simulink model "AccTarSel"  (R2018b)
settings: Solver=FixedStepDiscrete  StartTime=0.0  StopTime=inf  FixedStep=0.01  RelTol=1e-3
PostLoadFcn:
  | if any(exist('dsrtsu_mdlpostloadfcn', 'file') ~= 0), dsrtsu_mdlpostloadfcn('Execute', bdroot); end
values from neighbouring files (symbols this model uses):
  P_adtMaxBDC = 1.0    [AccTarSel.sldd]
  P_aFOCApproachIntpAcitve = -0.6    [AccTarSel.sldd]
  P_aFOCApproachIntpEnsure = -1.8    [AccTarSel.sldd]
  P_CutInEnable = 1.0    [AccTarSel.sldd]
  P_dAimMin = 4.5    [AccTarSel.sldd]
  P_dAimMinAVP = 1.5    [AccTarSel.sldd]
  P_dObjDrvOffMax = 5.0    [AccTarSel.sldd]
  P_dObjDrvOffMin = 3.0    [AccTarSel.sldd]
  P_dObjLowHystDecToStop = 4.5    [AccTarSel.sldd]
  P_dObjLowHystDecToStopAVP = 1.5    [AccTarSel.sldd]
  P_dObjUpperHystDecToStop = 5.0    [AccTarSel.sldd]
  P_dResMax = 5.0    [AccTarSel.sldd]
  P_dStandStill = 3.0    [AccTarSel.sldd]
  P_dStandStillMin = 2.0    [AccTarSel.sldd]
  P_dvarYMax4PO = 1.0    [AccTarSel.sldd]
  P_dyCutInThres = 3.6    [AccTarSel.sldd]
  P_facBDCInit = 0.7    [AccTarSel.sldd]
  P_facBDCIterCalc = 0.8    [AccTarSel.sldd]
  P_facFOCNegDiff = 0.3    [AccTarSel.sldd]
  P_facFOCPosDiff = 0.2    [AccTarSel.sldd]
  P_kapHystThres = 0.0005    [AccTarSel.sldd]
  P_PlausIntegDisable = 0.0    [AccTarSel.sldd]
  P_plausMin4PO = 0.5    [AccTarSel.sldd]
  P_probExistMin4PO = 0.8    [AccTarSel.sldd]
  P_StandObjEnable = 0.0    [AccTarSel.sldd]
  P_tAxTrackNegLower = 0.3    [AccTarSel.sldd]
  P_tAxTrackNegUpper = 0.6    [AccTarSel.sldd]
  P_tAxTrackPosLower = 1.0    [AccTarSel.sldd]
  P_tAxTrackPosUpper = 2.0    [AccTarSel.sldd]
  P_tBDCStartFilt = 0.2    [AccTarSel.sldd]
  P_tCSC = 3.5    [AccTarSel.sldd]
  P_tCurvFilt = 0.2    [AccTarSel.sldd]
  P_tCutInFilt = 0.5    [AccTarSel.sldd]
  P_tFiltAxAbsPONegFast = 0.1    [AccTarSel.sldd]
  P_tFiltAxAbsPONegSlow = 0.4    [AccTarSel.sldd]
  P_tFiltAxAbsPOPosFast = 1.2    [AccTarSel.sldd]
  P_tFiltAxAbsPOPosSlow = 2.0    [AccTarSel.sldd]
  P_tFiltAxAbsPOStand = 2.0    [AccTarSel.sldd]
  P_tFiltDAim = 0.1    [AccTarSel.sldd]
  P_tFiltDsd = 0.1    [AccTarSel.sldd]
  P_tFiltSpdLim = 3.0    [AccTarSel.sldd]
  P_tFiltVxAxPOFast = 0.15    [AccTarSel.sldd]
  P_tFiltVxAxPOSlow = 0.25    [AccTarSel.sldd]
  P_tFOCStatAccelFast = 4.0    [AccTarSel.sldd]
  P_tFOCStatAccelSlow = 3.5    [AccTarSel.sldd]
  P_tFOCStatDecelFast = 4.0    [AccTarSel.sldd]
  P_tFOCStatDecelSlow = 3.2    [AccTarSel.sldd]
  P_tMinDrvPhase = 2.0    [AccTarSel.sldd]
  P_tPredObjLeav = 1.2    [AccTarSel.sldd]
  P_tRollingFilt = 0.5    [AccTarSel.sldd]
  P_tRollingFinFilt = 1.0    [AccTarSel.sldd]
  P_tSSCNeg = 4.5    [AccTarSel.sldd]
  P_tSSCPos = 5.5    [AccTarSel.sldd]
  P_tToStop = 5.0    [AccTarSel.sldd]
  P_tToStopInBDC = 6.0    [AccTarSel.sldd]
  P_tToStopTrig = 4.0    [AccTarSel.sldd]
  P_vEgoDecToStop = 3.0    [AccTarSel.sldd]
  P_vEgoLowBDC = 4.0    [AccTarSel.sldd]
  P_vFOCNegDiff = 4.0    [AccTarSel.sldd]
  P_vFOCPosDiff = 5.0    [AccTarSel.sldd]
  P_vFOCStationaryFast = 15.0    [AccTarSel.sldd]
  P_vFOCStationarySlow = 5.0    [AccTarSel.sldd]
  P_vObjDrvOff = 0.5    [AccTarSel.sldd]
  P_vObjLowHystDecToStop = 0.5    [AccTarSel.sldd]
  P_vObjNoStop = 1.0    [AccTarSel.sldd]
  P_vObjReCalc = 1.0    [AccTarSel.sldd]
  P_vObjStop = 0.3    [AccTarSel.sldd]
  P_vObjUpperHystDecToStop = 0.8    [AccTarSel.sldd]
  P_vStandStill = 0.3    [AccTarSel.sldd]
  P_vStandStillHyst = 0.3    [AccTarSel.sldd]
  P_vyCutInThres = 0.5    [AccTarSel.sldd]
libraries: simulink x21, LPFilter x12
(part 5 of 11)

== system AccTarSel/calcCancelFlag/If Action Subsystem1 ==
  SYS_Info : Inport
  HoldTimeK1 : Inport  Port=2
  Action Port : ActionPort  ActionType=elseif
  Add : Sum  Inputs=+-
  Bus Selector : BusSelector  OutputSignals=dT
  Constant : Constant  OutDataTypeStr=boolean
  Constant1 : Constant  Value=0  OutDataTypeStr=single
  Max : MinMax  Function=max  Inputs=2
  CancelFlag : Outport
  HoldTime : Outport  Port=2
  wires:
  Max/1 -> HoldTime/1
  Constant/1 -> CancelFlag/1
  SYS_Info/1 -> Bus Selector/1
  HoldTimeK1/1 -> Add/1
  Bus Selector/1 -> Add/2  "<dT>"
  Add/1 -> Max/1
  Constant1/1 -> Max/2

== system AccTarSel/calcCancelFlag/If Action Subsystem2 ==
  Action Port : ActionPort  ActionType=else
  Constant : Constant  Value=0  OutDataTypeStr=boolean
  Constant1 : Constant  Value=0  OutDataTypeStr=single
  CancelFlag : Outport
  HoldTime : Outport  Port=2
  wires:
  Constant/1 -> CancelFlag/1
  Constant1/1 -> HoldTime/1

== system AccTarSel/ACC_Control/AccelBoundCtrl/LowerLimitation ==
  note: expand lower limitation according to:
      | vehicle speed
      | slope
  Constant : Constant  Value=-5  OutDataTypeStr=single
  Out1 : Outport
  wires:
  Constant/1 -> Out1/1

== system AccTarSel/ACC_Control/AccelBoundCtrl/UpperLimitation ==
  note: expand lower limitation according to:
      | vehicle speed
      | slope
      | engine capacity
  Constant : Constant  Value=2  OutDataTypeStr=single
  Out1 : Outport
  wires:
  Constant/1 -> Out1/1

== system AccTarSel/ACC_Control/ArbitraryMix/Subsystem ==
  aCvArray : Inport
  numASrc : Inport  Port=2
  Add : Sum
  Constant : Constant  Value=0  OutDataTypeStr=int32
  Constant1 : Constant  Value=16  OutDataTypeStr=single
  Constant2 : Constant  OutDataTypeStr=int32
  For Iterator : ForIterator  IterationSource=external  IndexMode=Zero-based
  Memory : Memory  InheritSampleTime=on
  Memory1 : Memory  InheritSampleTime=on
  Relational Operator : RelationalOperator  Operator===  OutDataTypeStr=boolean  RndMeth=Simplest
  Relational Operator1 : RelationalOperator  Operator=<  OutDataTypeStr=boolean  RndMeth=Simplest
  Selector : Selector  IndexMode=Zero-based  InputPortWidth=4  IndexOptions=Index vector (port)  Indices=[1 3]  OutputSizes=1
  Switch : Switch  Criteria=u2 > Threshold
  Switch1 : Switch  Criteria=u2 > Threshold
  Switch2 : Switch  Criteria=u2 > Threshold
  aMin : Outport
  CMDType : Outport  Port=2
  wires:
  numASrc/1 -> For Iterator/1
  For Iterator/1 -> Selector/2, Add/1, Relational Operator/1
  Constant/1 -> Relational Operator/2
  Relational Operator/1 -> Switch/2
  Constant1/1 -> Switch/1
  aCvArray/1 -> Selector/1
  Selector/1 -> Switch1/1, Relational Operator1/1
  Switch/1 -> Switch1/3, Relational Operator1/2
  Memory/1 -> Switch/3
  Relational Operator1/1 -> Switch1/2, Switch2/2
  Switch1/1 -> aMin/1, Memory/1
  Switch2/1 -> Memory1/1, CMDType/1
  Memory1/1 -> Switch2/3
  Constant2/1 -> Add/2
  Add/1 -> Switch2/1

== system AccTarSel/ACC_Control/ArbitraryMix/calcAFOC ==
  FOCInfo : Inport
  Constant2 : Constant  Value=6  OutDataTypeStr=int32
  For Iterator Subsystem : Subsystem  TreatAsAtomicUnit=on
  Min : MinMax
  OR : Logic  Operator=OR  Inputs=1  AllPortsSameDT=off  OutDataTypeStr=boolean
  aFOC : Outport
  DecToStop : Outport  Port=2
  wires:
  Min/1 -> aFOC/1
  FOCInfo/1 -> For Iterator Subsystem/2(FOCInfo)
  For Iterator Subsystem/1(aFOCArray) -> Min/1
  For Iterator Subsystem/2(DecToStopArray) -> OR/1
  OR/1 -> DecToStop/1
  Constant2/1 -> For Iterator Subsystem/1(numFOC)

== system AccTarSel/ACC_Control/FollowObjCtrl/FollowObjInvalid ==
  Action Port : ActionPort  ActionType=else
  Constant : Constant  Value=16  OutDataTypeStr=single
  Constant1 : Constant  Value=0  OutDataTypeStr=boolean
  Constant{3..8,10} (7 alike) : Constant  Value=0  OutDataTypeStr=single
  Constant2 : Constant  OutDataTypeStr=boolean
  Constant9 : Constant  Value=0  OutDataTypeStr=boolean
  a : Outport
  DecToStop : Outport  Port=2
  FirstCyc : Outport  Port=3  InitialOutput=0
  dAim : Outport  Port=4  InitialOutput=0
  aStat : Outport  Port=5  InitialOutput=0
  aApproach : Outport  Port=6  InitialOutput=0
  ApproachCase : Outport  Port=7  InitialOutput=0
  tObjStop : Outport  Port=8  InitialOutput=0
  dSlowDown : Outport  Port=9  InitialOutput=0
  ObjLeaving : Outport  Port=10  InitialOutput=0
  dImmerseAdj : Outport  Port=11  InitialOutput=0
  wires:
  Constant/1 -> a/1
  Constant1/1 -> DecToStop/1
  Constant2/1 -> FirstCyc/1
  Constant3/1 -> dAim/1
  Constant4/1 -> aStat/1
  Constant5/1 -> aApproach/1
  Constant6/1 -> ApproachCase/1
  Constant7/1 -> tObjStop/1
  Constant8/1 -> dSlowDown/1
  Constant9/1 -> ObjLeaving/1
  Constant10/1 -> dImmerseAdj/1

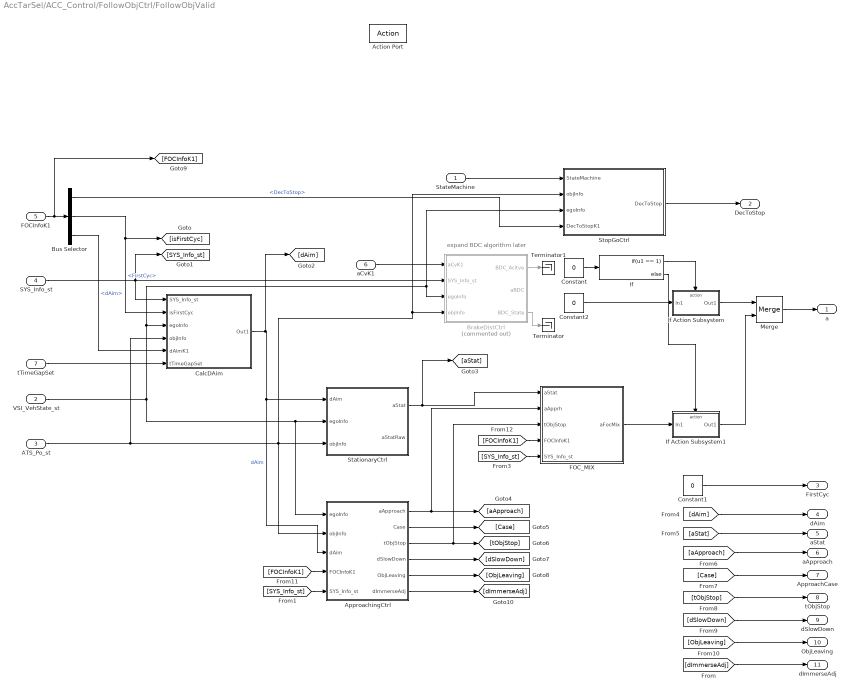
== system AccTarSel/ACC_Control/FollowObjCtrl/FollowObjValid ==
  note: expand BDC algorithm later
  StateMachine : Inport
  VSI_VehState_st : Inport  Port=2
  ATS_Po_st : Inport  Port=3
  SYS_Info_st : Inport  Port=4
  FOCInfoK1 : Inport  Port=5
  aCvK1 : Inport  Port=6
  tTimeGapSet : Inport  Port=7
  Action Port : ActionPort  ActionType=then
  ApproachingCtrl : Subsystem
  BrakeDistCtrl : Subsystem  Commented=on
  Bus Selector : BusSelector  OutputSignals=DecToStop,FirstCyc,dAim
  CalcDAim : Subsystem
  Constant : Constant  Value=0  OutDataTypeStr=boolean
  Constant1 : Constant  Value=0  OutDataTypeStr=boolean
  Constant2 : Constant  Value=0  OutDataTypeStr=single
  FOC_MIX : Subsystem
  If : If  IfExpression=u1 == 1
  If Action Subsystem : Subsystem  TreatAsAtomicUnit=on
  If Action Subsystem1 : Subsystem  TreatAsAtomicUnit=on
  Merge : Merge  InitialOutput=0
  StationaryCtrl : Subsystem
  StopGoCtrl : Subsystem
  Terminator : Terminator
  Terminator1 : Terminator
  a : Outport  InitialOutput=0
  DecToStop : Outport  Port=2  InitialOutput=0
  FirstCyc : Outport  Port=3  InitialOutput=0
  dAim : Outport  Port=4  InitialOutput=0
  aStat : Outport  Port=5  InitialOutput=0
  aApproach : Outport  Port=6  InitialOutput=0
  ApproachCase : Outport  Port=7  InitialOutput=0
  tObjStop : Outport  Port=8  InitialOutput=0
  dSlowDown : Outport  Port=9  InitialOutput=0
  ObjLeaving : Outport  Port=10  InitialOutput=0
  dImmerseAdj : Outport  Port=11  InitialOutput=0
  wires:
  ATS_Po_st/1 -> CalcDAim/4(objInfo), StopGoCtrl/2(objInfo), BrakeDistCtrl/4(objInfo), ApproachingCtrl/2(objInfo), StationaryCtrl/3(objInfo)
  CalcDAim/1(Out1) -> [dAim], ApproachingCtrl/3(dAim), StationaryCtrl/1(dAim)  "dAim"
  VSI_VehState_st/1 -> StopGoCtrl/3(egoInfo), BrakeDistCtrl/3(egoInfo), CalcDAim/3(egoInfo), ApproachingCtrl/1(egoInfo), StationaryCtrl/2(egoInfo)
  StationaryCtrl/1(aStat) -> [aStat], FOC_MIX/1(aStat)
  ApproachingCtrl/1(aApproach) -> [aApproach], FOC_MIX/2(aApprh)
  Constant/1 -> If/1
  FOC_MIX/1(aFocMix) -> If Action Subsystem1/1(In1)
  If/1 -> If Action Subsystem/Action
  If/2 -> If Action Subsystem1/Action
  If Action Subsystem/1(Out1) -> Merge/1
  If Action Subsystem1/1(Out1) -> Merge/2
  Merge/1 -> a/1
  StopGoCtrl/1(DecToStop) -> DecToStop/1
  FOCInfoK1/1 -> [FOCInfoK1], Bus Selector/1
  BrakeDistCtrl/3(BDC_State) -> Terminator/1
  SYS_Info_st/1 -> [SYS_Info_st], CalcDAim/1(SYS_Info_st), BrakeDistCtrl/2(SYS_Info_st)
  aCvK1/1 -> BrakeDistCtrl/1(aCvK1)
  Constant1/1 -> FirstCyc/1
  Bus Selector/2 -> CalcDAim/2(isFirstCyc), [isFirstCyc]  "<FirstCyc>"
  [FOCInfoK1] -> ApproachingCtrl/4(FOCInfoK1)
  [SYS_Info_st] -> ApproachingCtrl/5(SYS_Info_st)
  tTimeGapSet/1 -> CalcDAim/6(tTimeGapSet)
  ApproachingCtrl/3(tObjStop) -> [tObjStop], FOC_MIX/3(tObjStop)
  [FOCInfoK1] -> FOC_MIX/4(FOCInfoK1)
  [SYS_Info_st] -> FOC_MIX/5(SYS_Info_st)
  [dAim] -> dAim/1
  [aStat] -> aStat/1
  ApproachingCtrl/2(Case) -> [Case]
  ApproachingCtrl/4(dSlowDown) -> [dSlowDown]
  ApproachingCtrl/5(ObjLeaving) -> [ObjLeaving]
  [aApproach] -> aApproach/1
  [Case] -> ApproachCase/1
  [tObjStop] -> tObjStop/1
  [dSlowDown] -> dSlowDown/1
  [ObjLeaving] -> ObjLeaving/1
  Bus Selector/1 -> StopGoCtrl/4(DecToStopK1)  "<DecToStop>"
  Bus Selector/3 -> CalcDAim/5(dAimK1)  "<dAim>"
  BrakeDistCtrl/1(BDC_Acitve) -> Terminator1/1
  Constant2/1 -> If Action Subsystem/1(In1)
  StateMachine/1 -> StopGoCtrl/1(StateMachine)
  ApproachingCtrl/6(dImmerseAdj) -> [dImmerseAdj]
  [dImmerseAdj] -> dImmerseAdj/1

== system AccTarSel/ACC_Control/OvertakeSuppression/If Action Subsystem ==
  note: Type:
      | 0	Unknown
      | 1	Pedestrain
      | 2	Bi/Motor cycle
      | 3	Bus
      | 4	Medium car
      | 5	Truck
      | 6	Three-wheel motor
      | 7	Special car
      | 8	Tiny car
      | 9	Ambluance
      | 10	Uncertain
  index : Inport
  TargetInfo : Inport  Port=2
  egoInfo : Inport  Port=3
  Action Port : ActionPort  ActionType=then
  AND : Logic  Inputs=4  AllPortsSameDT=off  OutDataTypeStr=boolean
  Add : Sum
  Bus Selector : BusSelector  OutputSignals=objdata_st
  Bus Selector1 : BusSelector  OutputSignals=vx,dx,Valid,Type
  Bus Selector2 : BusSelector  OutputSignals=vRef
  Constant : Constant  Value=40  OutDataTypeStr=single
  Constant1 : Constant  Value=30  OutDataTypeStr=single
  Constant2 : Constant  Value=0  OutDataTypeStr=single
  Constant3 : Constant  Value=3  OutDataTypeStr=single
  Constant4 : Constant  Value=5  OutDataTypeStr=single
  OR : Logic  Operator=OR  AllPortsSameDT=off  OutDataTypeStr=boolean
  Relational Operator : RelationalOperator  Operator=<=  OutDataTypeStr=boolean  RndMeth=Simplest
  Relational Operator1 : RelationalOperator  OutDataTypeStr=boolean  RndMeth=Simplest
  Relational Operator2 : RelationalOperator  Operator===  OutDataTypeStr=boolean  RndMeth=Simplest
  Relational Operator3 : RelationalOperator  Operator===  OutDataTypeStr=boolean  RndMeth=Simplest
  Selector1 : Selector  IndexMode=Zero-based  InputPortWidth=40  IndexOptions=Index vector (port)  Indices=[1 3]  OutputSizes=1
  Switch : Switch  Criteria=u2 > Threshold
  Out1 : Outport
  wires:
  TargetInfo/1 -> Bus Selector/1
  Bus Selector/1 -> Selector1/1  "<objdata_st>"
  index/1 -> Selector1/2
  Selector1/1 -> Bus Selector1/1  "ObjData"
  Bus Selector1/2 -> Relational Operator1/1, Relational Operator/1  "<dx>"
  Constant1/1 -> Relational Operator/2
  Constant2/1 -> Relational Operator1/2
  Relational Operator1/1 -> AND/1
  Relational Operator/1 -> AND/2
  Bus Selector1/3 -> AND/3  "<Valid>"
  AND/1 -> Switch/2
  Bus Selector1/1 -> Add/2  "<vx>"
  egoInfo/1 -> Bus Selector2/1
  Bus Selector2/1 -> Add/1  "<vRef>"
  Add/1 -> Switch/1
  Constant/1 -> Switch/3
  Switch/1 -> Out1/1
  Bus Selector1/4 -> Relational Operator3/1, Relational Operator2/1  "<Type>"
  Constant3/1 -> Relational Operator2/2
  Constant4/1 -> Relational Operator3/2
  Relational Operator2/1 -> OR/1
  Relational Operator3/1 -> OR/2
  OR/1 -> AND/4

== system AccTarSel/ACC_Control/OvertakeSuppression/If Action Subsystem1 ==
  Action Port : ActionPort  ActionType=else
  Constant : Constant  Value=40  OutDataTypeStr=single
  Out1 : Outport
  wires:
  Constant/1 -> Out1/1

== system AccTarSel/ACC_Control/OvertakeSuppression/If Action Subsystem2 ==
  note: Type:
      | 0	Unknown
      | 1	Pedestrain
      | 2	Bi/Motor cycle
      | 3	Bus
      | 4	Medium car
      | 5	Truck
      | 6	Three-wheel motor
      | 7	Special car
      | 8	Tiny car
      | 9	Ambluance
      | 10	Uncertain
  index : Inport
  TargetInfo : Inport  Port=2
  egoInfo : Inport  Port=3
  Action Port : ActionPort  ActionType=then
  AND : Logic  Inputs=4  AllPortsSameDT=off  OutDataTypeStr=boolean
  Add : Sum
  Bus Selector : BusSelector  OutputSignals=objdata_st
  Bus Selector1 : BusSelector  OutputSignals=vx,dx,Valid,Type
  Bus Selector2 : BusSelector  OutputSignals=vRef
  Constant : Constant  Value=40  OutDataTypeStr=single
  Constant1 : Constant  Value=30  OutDataTypeStr=single
  Constant2 : Constant  Value=0  OutDataTypeStr=single
  Constant3 : Constant  Value=3  OutDataTypeStr=single
  Constant4 : Constant  Value=5  OutDataTypeStr=single
  OR : Logic  Operator=OR  AllPortsSameDT=off  OutDataTypeStr=boolean
  Relational Operator : RelationalOperator  Operator=<=  OutDataTypeStr=boolean  RndMeth=Simplest
  Relational Operator1 : RelationalOperator  OutDataTypeStr=boolean  RndMeth=Simplest
  Relational Operator2 : RelationalOperator  Operator===  OutDataTypeStr=boolean  RndMeth=Simplest
  Relational Operator3 : RelationalOperator  Operator===  OutDataTypeStr=boolean  RndMeth=Simplest
  Selector1 : Selector  IndexMode=Zero-based  InputPortWidth=40  IndexOptions=Index vector (port)  Indices=[1 3]  OutputSizes=1
  Switch : Switch  Criteria=u2 > Threshold
  Out1 : Outport
  wires:
  TargetInfo/1 -> Bus Selector/1
  Bus Selector/1 -> Selector1/1  "<objdata_st>"
  index/1 -> Selector1/2
  Selector1/1 -> Bus Selector1/1  "ObjData"
  Bus Selector1/2 -> Relational Operator/1, Relational Operator1/1  "<dx>"
  Constant1/1 -> Relational Operator/2
  Constant2/1 -> Relational Operator1/2
  Relational Operator1/1 -> AND/1
  Relational Operator/1 -> AND/2
  Bus Selector1/3 -> AND/3  "<Valid>"
  AND/1 -> Switch/2
  Bus Selector1/1 -> Add/2  "<vx>"
  egoInfo/1 -> Bus Selector2/1
  Bus Selector2/1 -> Add/1  "<vRef>"
  Add/1 -> Switch/1
  Constant/1 -> Switch/3
  Switch/1 -> Out1/1
  Bus Selector1/4 -> Relational Operator3/1, Relational Operator2/1  "<Type>"
  Constant3/1 -> Relational Operator2/2
  Constant4/1 -> Relational Operator3/2
  Relational Operator2/1 -> OR/1
  Relational Operator3/1 -> OR/2
  OR/1 -> AND/4

== system AccTarSel/ACC_Control/OvertakeSuppression/If Action Subsystem3 ==
  Action Port : ActionPort  ActionType=else
  Constant : Constant  Value=40  OutDataTypeStr=single
  Out1 : Outport
  wires:
  Constant/1 -> Out1/1

== system AccTarSel/ACC_Control/SetSpdCtrl/If Action Subsystem ==
  In1 : Inport
  Action Port : ActionPort  ActionType=then
  Out1 : Outport
  wires:
  In1/1 -> Out1/1

== system AccTarSel/ACC_Control/SetSpdCtrl/If Action Subsystem1 ==
  In1 : Inport
  Action Port : ActionPort  ActionType=else
  Out1 : Outport
  wires:
  In1/1 -> Out1/1

== system AccTarSel/ACC_Target_Selection/Subsystem/ValidObjCalc ==
  objInfo : Inport
  In2 : Inport  Port=2
  In3 : Inport  Port=3
  ATS_Internal_K1 : Inport  Port=4
  SYS_Info_st : Inport  Port=5
  Bus Creator : BusCreator  Inputs=12  OutDataTypeStr=Bus: ATS_OBJINFO_ST  NonVirtualBus=on
  Bus Selector : BusSelector  OutputSignals=dx,dy,vx,vy,ID
  CutInCalc : Subsystem
  EgoCourseDeviation : Subsystem
  LanePlausCalc : Subsystem
  LaneProbCalc : Subsystem
  TargetPlausCheck : Subsystem
  isTargetValid : Outport
  "ats_objInfo " : Outport  Port=2
  wires:
  objInfo/1 -> Bus Selector/1, LanePlausCalc/3(objInfo), CutInCalc/1(objInfo), LaneProbCalc/1(objInfo), TargetPlausCheck/1(In1), EgoCourseDeviation/1(objInfo)
  In2/1 -> EgoCourseDeviation/2(egoTrajLane_st)  "egoTrajLane_st"
  LaneProbCalc/1(Out1) -> LanePlausCalc/1(probEgoLane), Bus Creator/9  "probEgoLane"
  CutInCalc/3(isCutIn) -> LanePlausCalc/2(isCutIn)
  EgoCourseDeviation/1(dyToTraj) -> CutInCalc/2(dyToTraj), LaneProbCalc/2(In2), Bus Creator/5
  LanePlausCalc/1(Out1) -> Bus Creator/10, TargetPlausCheck/2(In2)  "plausEgoLane"
  In3/1 -> TargetPlausCheck/3(In3)  "VSI_VehState_st"
  TargetPlausCheck/1(Out1) -> Bus Creator/11, isTargetValid/1  "ValidEgoLane"
  Bus Selector/1 -> Bus Creator/1  "<dx>"
  Bus Selector/2 -> Bus Creator/2  "<dy>"
  Bus Creator/1 -> "ats_objInfo "/1
  CutInCalc/1(dyCutInPred) -> Bus Creator/6  "dyCutInPred"
  Bus Selector/3 -> Bus Creator/3  "<vx>"
  Bus Selector/4 -> Bus Creator/4  "<vy>"
  ATS_Internal_K1/1 -> LanePlausCalc/4(ATS_Internal_K1), LaneProbCalc/3(ATS_Internal_K1), CutInCalc/3(ATS_Internal_K1)
  Bus Selector/5 -> Bus Creator/12  "<ID>"
  SYS_Info_st/1 -> LanePlausCalc/5(SYS_Info_st), CutInCalc/4(SYS_Info_st)
  CutInCalc/2(probCutInFilt) -> Bus Creator/8  "probCutInFilt"
  CutInCalc/4(probCutInRaw) -> Bus Creator/7  "probCutInRaw"

== system AccTarSel/ACC_Target_Selection/TargetSel/If Action Subsystem ==
  In1 : Inport
  In2 : Inport  Port=2
  Action Port : ActionPort  ActionType=then
  Bus Selector : BusSelector  OutputSignals=dx,dy,vx,vy,ax,Type,MotionSts
  Constant : Constant  OutDataTypeStr=boolean
  valid : Outport
  index : Outport  Port=2
  dx : Outport  Port=3
  dy : Outport  Port=4
  vx : Outport  Port=5
  vy : Outport  Port=6
  ax : Outport  Port=7
  Type : Outport  Port=8
  MotionSts : Outport  Port=9
  wires:
  In1/1 -> Bus Selector/1
  Bus Selector/1 -> dx/1  "<dx>"
  Bus Selector/2 -> dy/1  "<dy>"
  Bus Selector/3 -> vx/1  "<vx>"
  Bus Selector/4 -> vy/1  "<vy>"
  Bus Selector/5 -> ax/1  "<ax>"
  In2/1 -> index/1
  Constant/1 -> valid/1
  Bus Selector/6 -> Type/1  "<Type>"
  Bus Selector/7 -> MotionSts/1  "<MotionSts>"

== system AccTarSel/ACC_Target_Selection/TargetSel/If Action Subsystem1 ==
  Action Port : ActionPort  ActionType=elseif
  Constant{,1..4,7..8} (7 alike) : Constant  Value=0  OutDataTypeStr=single
  Constant5 : Constant  Value=255  OutDataTypeStr=single
  Constant6 : Constant  Value=0  OutDataTypeStr=boolean
  valid : Outport
  index : Outport  Port=2
  dx : Outport  Port=3
  dy : Outport  Port=4
  vx : Outport  Port=5
  vy : Outport  Port=6
  ax : Outport  Port=7
  Type : Outport  Port=8
  MotionSts : Outport  Port=9
  wires:
  Constant/1 -> dx/1
  Constant1/1 -> dy/1
  Constant2/1 -> vx/1
  Constant3/1 -> vy/1
  Constant4/1 -> ax/1
  Constant5/1 -> index/1
  Constant6/1 -> valid/1
  Constant7/1 -> Type/1
  Constant8/1 -> MotionSts/1

== system AccTarSel/AVP_Simu/calcAVPInfo/dxPredict ==
  dxSet : Inport
  egoInfo : Inport  Port=2
  SYS_Info : Inport  Port=3
  Add : Sum
  Add1 : Sum  Inputs=+-
  Bus Selector : BusSelector  OutputSignals=vRef,aRef
  Bus Selector1 : BusSelector  OutputSignals=dT
  Constant : Constant  Value=0.1  OutDataTypeStr=single
  Max : MinMax  Function=max  Inputs=2
  Memory : Memory
  Memory1 : Memory
  Multiply : Product
  Multiply1 : Product
  Relational Operator : RelationalOperator  Operator=~=  OutDataTypeStr=boolean  RndMeth=Simplest
  Square : Math  Operator=square  SaturateOnIntegerOverflow=on
  Switch1 : Switch  Criteria=u2 > Threshold
  dxPredict : Outport
  wires:
  dxSet/1 -> Switch1/1, Relational Operator/1, Memory/1
  Relational Operator/1 -> Switch1/2
  Memory/1 -> Relational Operator/2
  egoInfo/1 -> Bus Selector/1
  Bus Selector/1 -> Multiply/1  "<vRef>"
  Bus Selector1/1 -> Square/1, Multiply/2  "<dT>"
  SYS_Info/1 -> Bus Selector1/1
  Bus Selector/2 -> Multiply1/1  "<aRef>"
  Square/1 -> Multiply1/2
  Multiply/1 -> Add/1
  Multiply1/1 -> Add/2
  Max/1 -> Memory1/1, dxPredict/1
  Memory1/1 -> Add1/1
  Add/1 -> Add1/2
  Add1/1 -> Switch1/3
  Switch1/1 -> Max/2
  Constant/1 -> Max/1

== system AccTarSel/EgoCourseFusion/CurvatureFilt/If Action Subsystem ==
  In1 : Inport
  Action Port : ActionPort  ActionType=then
  Out1 : Outport
  wires:
  In1/1 -> Out1/1

== system AccTarSel/EgoCourseFusion/CurvatureFilt/If Action Subsystem1 ==
  In1 : Inport
  Action Port : ActionPort  ActionType=else
  Out1 : Outport
  wires:
  In1/1 -> Out1/1

== system AccTarSel/ObjAdapter/For Each Subsystem/calcDx ==
  note: half length
  note: mass center
  note: rear axls to front bumper
  <longPosition> : Inport
  <length> : Inport  Port=2
  Add : Sum  Inputs=+--
  Constant1 : Constant  Value=3.68  OutDataTypeStr=single
  Gain : Gain  Gain=0.5
  dx : Outport
  wires:
  <longPosition>/1 -> Add/1
  Add/1 -> dx/1  "dx"
  <length>/1 -> Gain/1
  Gain/1 -> Add/2
  Constant1/1 -> Add/3
